simulink library "SpeedgoatModified"  (R2013a)
settings: Solver=ode45  StartTime=0.0  StopTime=60  RelTol=1e-3
undefined symbols (not defined in the file): standard
libraries: speedgoatlib x25, xpcseriallib x6, simulink x4, xpclib x2
settings Model: Creator=bgbuss  LastModifiedBy=bgbuss

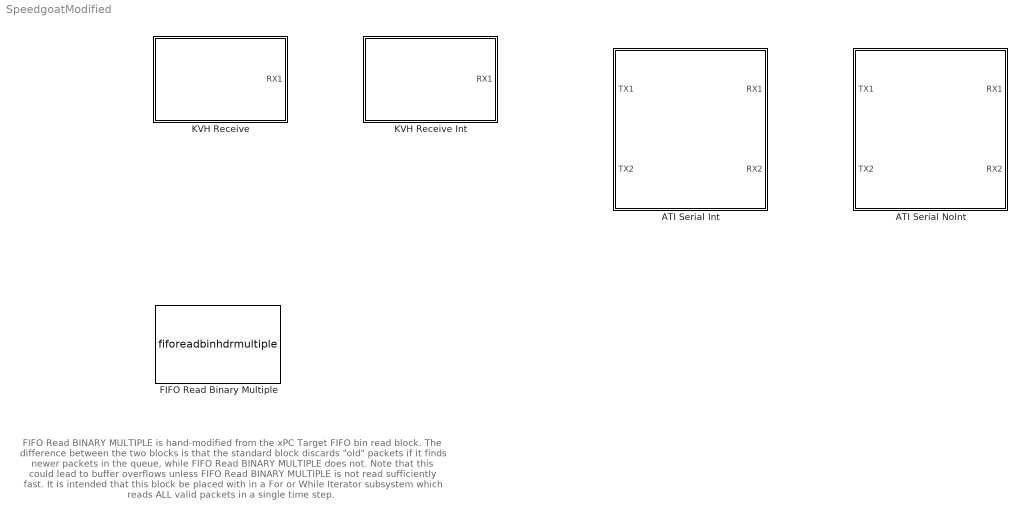
== system SpeedgoatModified ==
  note: FIFO Read BINARY MULTIPLE is hand-modified from the
      | xPC Target FIFO bin read block. The difference between the
      | two blocks is that the standard block discards "old" packets if it
      | finds newer packets in the queue, while FIFO Read BINARY MULTIPLE
      | does not. Note that this could lead to buffer overflows unless FIFO Read
      | BINARY MULTIPLE is not read sufficiently fast. It is intended that this block
      | be placed with in a For or While Iterator subsystem which reads ALL valid
      | packets in a single time step.
  ATI Serial Int : Subsystem
      mask Display:
      | disp('IO503\nTPMC466\nSend Interrupt-Free\nReceive Interrup-Driven')
      | 
      | port_label('input', 1, 'TX1')
      | port_label('input', 2, 'TX2')
      | 
      | port_label('output', 1, 'RX1')
      | port_label('output', 2, 'RX2')
  ATI Serial NoInt : Subsystem
      mask Display:
      | disp('IO503\nTPMC466\nSend Interrupt-Free\nReceive Interrup-Free')
      | 
      | port_label('input', 1, 'TX1')
      | port_label('input', 2, 'TX2')
      | 
      | port_label('output', 1, 'RX1')
      | port_label('output', 2, 'RX2')
  FIFO Read Binary Multiple : S-Function  FunctionName=fiforeadbinhdrmultiple  Parameters=maxsize, outputtype, sampletime, hdr, hlengths, lengths, hold, enable  EnableBusSupport=off  mask(Asynchronous FIFO Block: reader){header={char([170, 1]), char([170,2])}, lengths=[3 4], hold=Zero output if no new data, enable=off, maxsize=1024, outputtype=8 bit uint null terminated, sampletime=0.01}
      mask prompts: lengths "Message Lengths:"; hold "Output behavior:"; enable "Enable input:"; maxsize "Maximum read size:"; outputtype "Output vector type:"
      mask help: FIFO read multiple binary headers
      mask init:
      | [maskdisplay, hdr, hlengths] = mfifobinhdrmultiple( header, lengths );
      | set_param( gcb, 'MaskDisplay', maskdisplay );
      mask Help: eval('xpcdoc(''FIFO_binread'')');
      mask TypeOptions hold: Hold last output if no new data | Zero output if no new data
      mask TypeOptions outputtype: count+32 bit int | count+32 bit uint | count+16 bit int | count+16 bit uint | 8 bit int null terminated | 8 bit uint null terminated
      mask Display: disp( 'FIFO Read\nBINARY MULTIPLE');port_label('input',1,'F');port_label('output',1,'1');port_label('output',2,'2');
  KVH Receive : Subsystem
      mask Display:
      | disp('IO503\nTPMC466\nReceive\nInterrup-Free')
      | port_label('output', 1, 'RX1')
  KVH Receive Int : Subsystem
      mask Display:
      | disp('IO503\nTPMC466\nReceive\nInterrup-Driven')
      | port_label('output', 1, 'RX1')

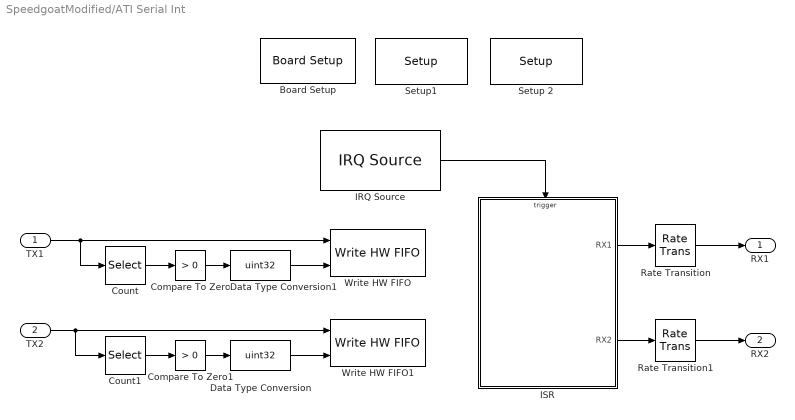
== system SpeedgoatModified/ATI Serial Int ==
  TX1 : Inport
  TX2 : Inport  Port=2
  Board Setup : speedgoatlib/IO503/TEWS TPMC466 Internal blocks/Board Setup  irqnum=5  slot=[4 4]
  Compare To Zero : simulink/Logic and Bit Operations/Compare To Zero  relop=>  OutDataTypeStr=uint8
  Compare To Zero1 : simulink/Logic and Bit Operations/Compare To Zero  relop=>  OutDataTypeStr=uint8
  Count : Selector  IndexMode=Zero-based  IndexOptions=Index vector (dialog)  Indices=0  OutputSizes=1
  Count1 : Selector  IndexMode=Zero-based  IndexOptions=Index vector (dialog)  Indices=0  OutputSizes=1
  Data Type Conversion : DataTypeConversion  OutDataTypeStr=uint32
  Data Type Conversion1 : DataTypeConversion  OutDataTypeStr=uint32
  IRQ Source : xpclib/Asynchronous Event/IRQ Source  irqNo=5  preempt=10  b_type=None/Other  slot=[4 4]
  ISR : Subsystem
  Rate Transition : RateTransition  Integrity=off  Deterministic=off
  Rate Transition1 : RateTransition  Integrity=off  Deterministic=off
  Setup 2 : speedgoatlib/IO503/TEWS TPMC466 Internal blocks/Setup   port=2  transceiver=RS485 half-duplex  standard=on  baudrate=1382400  bauddivisor=1  mode8x=16x (standard)  prescale=off  width=8  nstop=1  parity=Even  rlevel=half full (32)  ctsmode=none  xonoff=none  xon=17  xoff=19  rs485mode=on  rs485delay=0  slot=[4 4]
  "Setup1 " : speedgoatlib/IO503/TEWS TPMC466 Internal blocks/Setup   port=1  transceiver=RS485 half-duplex  standard=on  baudrate=1382400  bauddivisor=1  mode8x=16x (standard)  prescale=off  width=8  nstop=1  parity=Even  rlevel=half full (32)  ctsmode=none  xonoff=none  xon=17  xoff=19  rs485mode=on  rs485delay=0  slot=[4 4]
  Write HW FIFO : speedgoatlib/IO503/TEWS TPMC466 Internal blocks/Write HW FIFO  port=1  slot=[4 4]
  Write HW FIFO1 : speedgoatlib/IO503/TEWS TPMC466 Internal blocks/Write HW FIFO  port=2  slot=[4 4]
  RX1 : Outport
  RX2 : Outport  Port=2
  wires:
  Data Type Conversion1/1 -> Write HW FIFO/2
  Data Type Conversion/1 -> Write HW FIFO1/2
  Rate Transition/1 -> RX1/1
  IRQ Source/1 -> ISR/Trigger
  ISR/1(RX1) -> Rate Transition/1
  Rate Transition1/1 -> RX2/1
  ISR/2(RX2) -> Rate Transition1/1
  TX1/1 -> Count/1, Write HW FIFO/1
  TX2/1 -> Count1/1, Write HW FIFO1/1
  Count/1 -> Compare To Zero/1
  Count1/1 -> Compare To Zero1/1
  Compare To Zero1/1 -> Data Type Conversion/1
  Compare To Zero/1 -> Data Type Conversion1/1

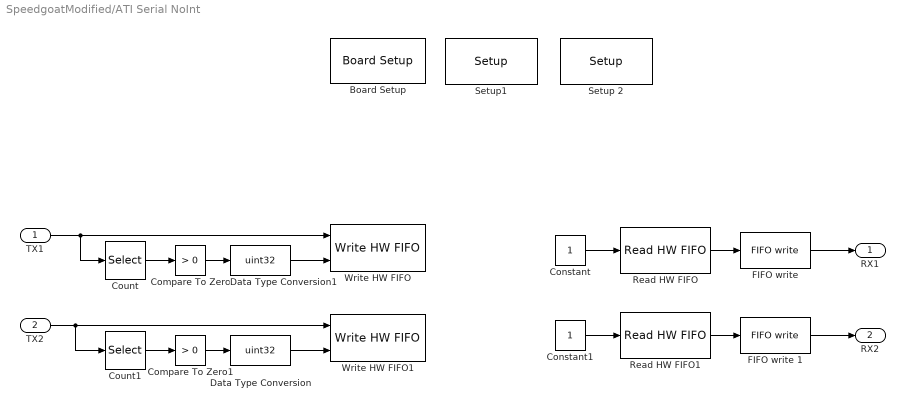
== system SpeedgoatModified/ATI Serial NoInt ==
  TX1 : Inport
  TX2 : Inport  Port=2
  Board Setup : speedgoatlib/IO503/TEWS TPMC466 Internal blocks/Board Setup  irqnum=5  slot=[4 4]
  Compare To Zero : simulink/Logic and Bit Operations/Compare To Zero  relop=>  OutDataTypeStr=uint8
  Compare To Zero1 : simulink/Logic and Bit Operations/Compare To Zero  relop=>  OutDataTypeStr=uint8
  Constant : Constant  OutDataTypeStr=Inherit: Inherit via back propagation
  Constant1 : Constant  OutDataTypeStr=Inherit: Inherit via back propagation
  Count : Selector  IndexMode=Zero-based  IndexOptions=Index vector (dialog)  Indices=0  OutputSizes=1
  Count1 : Selector  IndexMode=Zero-based  IndexOptions=Index vector (dialog)  Indices=0  OutputSizes=1
  Data Type Conversion : DataTypeConversion  OutDataTypeStr=uint32
  Data Type Conversion1 : DataTypeConversion  OutDataTypeStr=uint32
  "FIFO write " : xpcseriallib/FIFO write   size=256  inputtype=count+32 bit uint  present=off  sampletime=-1  id=IO503: IRQ 5 PCI Bus 4 Slot 4 (ATI F/T) 1
  FIFO write 1 : xpcseriallib/FIFO write   size=256  inputtype=count+32 bit uint  present=off  sampletime=-1  id=IO503: IRQ 5 PCI Bus 4 Slot 4 (ATI F/T) 2
  Read HW FIFO : speedgoatlib/IO503/TEWS TPMC466 Internal blocks/Read HW FIFO  port=1  flush=off  slot=[4 4]
  Read HW FIFO1 : speedgoatlib/IO503/TEWS TPMC466 Internal blocks/Read HW FIFO  port=2  flush=off  slot=[4 4]
  Setup 2 : speedgoatlib/IO503/TEWS TPMC466 Internal blocks/Setup   port=2  transceiver=RS485 half-duplex  standard=on  baudrate=1382400  bauddivisor=1  mode8x=16x (standard)  prescale=off  width=8  nstop=1  parity=Even  rlevel=almost full (56)  ctsmode=none  xonoff=none  xon=17  xoff=19  rs485mode=on  rs485delay=0  slot=[4 4]
  "Setup1 " : speedgoatlib/IO503/TEWS TPMC466 Internal blocks/Setup   port=1  transceiver=RS485 half-duplex  standard=on  baudrate=1382400  bauddivisor=1  mode8x=16x (standard)  prescale=off  width=8  nstop=1  parity=Even  rlevel=almost full (56)  ctsmode=none  xonoff=none  xon=17  xoff=19  rs485mode=on  rs485delay=0  slot=[4 4]
  Write HW FIFO : speedgoatlib/IO503/TEWS TPMC466 Internal blocks/Write HW FIFO  port=1  slot=[4 4]
  Write HW FIFO1 : speedgoatlib/IO503/TEWS TPMC466 Internal blocks/Write HW FIFO  port=2  slot=[4 4]
  RX1 : Outport  SourceOfInitialOutputValue=Input signal
  RX2 : Outport  Port=2  SourceOfInitialOutputValue=Input signal
  wires:
  Compare To Zero/1 -> Data Type Conversion1/1
  Compare To Zero1/1 -> Data Type Conversion/1
  Count1/1 -> Compare To Zero1/1
  Count/1 -> Compare To Zero/1
  TX2/1 -> Write HW FIFO1/1, Count1/1
  TX1/1 -> Write HW FIFO/1, Count/1
  Data Type Conversion/1 -> Write HW FIFO1/2
  Data Type Conversion1/1 -> Write HW FIFO/2
  Read HW FIFO1/1 -> FIFO write 1/1
  Constant1/1 -> Read HW FIFO1/1
  FIFO write 1/1 -> RX2/1
  Read HW FIFO/1 -> "FIFO write "/1
  Constant/1 -> Read HW FIFO/1
  "FIFO write "/1 -> RX1/1

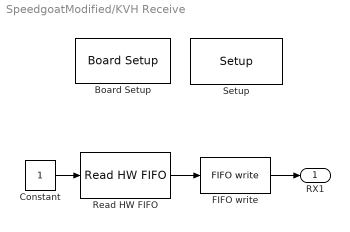
== system SpeedgoatModified/KVH Receive ==
  Board Setup : speedgoatlib/IO503/TEWS TPMC466 Internal blocks/Board Setup  irqnum=9  slot=[4 5]
  Constant : Constant  OutDataTypeStr=uint32
  "FIFO write " : xpcseriallib/FIFO write   size=256  inputtype=count+32 bit uint  present=off  sampletime=-1  id=IO503: IRQ 9 PCI Bus 4 Slot 5 (KVH IMU)
  Read HW FIFO : speedgoatlib/IO503/TEWS TPMC466 Internal blocks/Read HW FIFO  port=1  flush=off  slot=[4 5]
  "Setup " : speedgoatlib/IO503/TEWS TPMC466 Internal blocks/Setup   port=1  transceiver=RS422  standard=on  baudrate=921600  bauddivisor=1  mode8x=16x (standard)  prescale=off  width=8  nstop=1  parity=None  rlevel=almost full (56)  ctsmode=none  xonoff=none  xon=17  xoff=19  rs485mode=off  rs485delay=0  slot=[4 5]
  RX1 : Outport
  wires:
  Read HW FIFO/1 -> "FIFO write "/1
  "FIFO write "/1 -> RX1/1
  Constant/1 -> Read HW FIFO/1

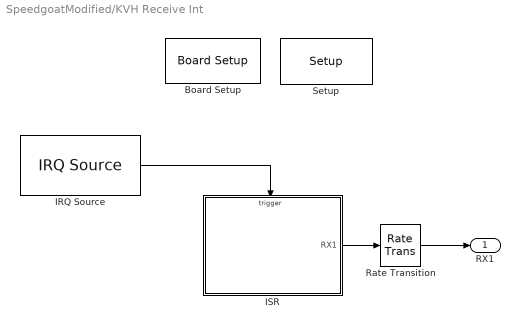
== system SpeedgoatModified/KVH Receive Int ==
  Board Setup : speedgoatlib/IO503/TEWS TPMC466 Internal blocks/Board Setup  irqnum=9  slot=[4 5]
  IRQ Source : xpclib/Asynchronous Event/IRQ Source  irqNo=9  preempt=10  b_type=None/Other  slot=[4 5]
  ISR : Subsystem
  Rate Transition : RateTransition  Integrity=off  Deterministic=off
  "Setup " : speedgoatlib/IO503/TEWS TPMC466 Internal blocks/Setup   port=1  transceiver=RS422  standard=on  baudrate=921600  bauddivisor=1  mode8x=16x (standard)  prescale=off  width=8  nstop=1  parity=None  rlevel=almost full (56)  ctsmode=none  xonoff=none  xon=17  xoff=19  rs485mode=off  rs485delay=0  slot=[4 5]
  RX1 : Outport
  wires:
  ISR/1(RX1) -> Rate Transition/1
  IRQ Source/1 -> ISR/Trigger
  Rate Transition/1 -> RX1/1

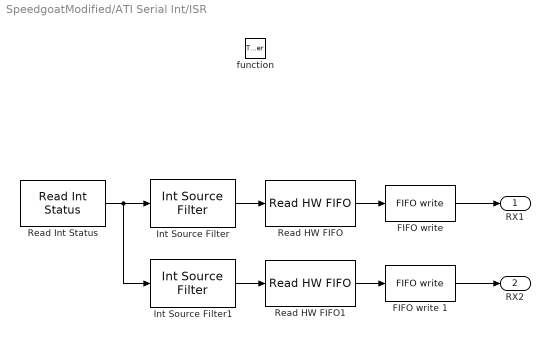
== system SpeedgoatModified/ATI Serial Int/ISR ==
  function : TriggerPort  TriggerType=function-call
  "FIFO write " : xpcseriallib/FIFO write   size=256  inputtype=count+32 bit uint  present=off  sampletime=-1  id=IO503: IRQ 5 PCI Bus 4 Slot 4 (ATI F/T) 1
  FIFO write 1 : xpcseriallib/FIFO write   size=256  inputtype=count+32 bit uint  present=off  sampletime=-1  id=IO503: IRQ 5 PCI Bus 4 Slot 4 (ATI F/T) 2
  Int Source Filter : speedgoatlib/IO503/TEWS TPMC466 Internal blocks/Int Source Filter  port=1  value=Receive data
  Int Source Filter1 : speedgoatlib/IO503/TEWS TPMC466 Internal blocks/Int Source Filter  port=2  value=Receive data
  Read HW FIFO : speedgoatlib/IO503/TEWS TPMC466 Internal blocks/Read HW FIFO  port=1  flush=off  slot=[4 4]
  Read HW FIFO1 : speedgoatlib/IO503/TEWS TPMC466 Internal blocks/Read HW FIFO  port=2  flush=off  slot=[4 4]
  Read Int Status : speedgoatlib/IO503/TEWS TPMC466 Internal blocks/Read Int Status  slot=[4 4]
  RX1 : Outport  SourceOfInitialOutputValue=Input signal
  RX2 : Outport  Port=2  SourceOfInitialOutputValue=Input signal
  wires:
  "FIFO write "/1 -> RX1/1
  Int Source Filter/1 -> Read HW FIFO/1
  Read Int Status/1 -> Int Source Filter1/1, Int Source Filter/1
  Read HW FIFO/1 -> "FIFO write "/1
  FIFO write 1/1 -> RX2/1
  Int Source Filter1/1 -> Read HW FIFO1/1
  Read HW FIFO1/1 -> FIFO write 1/1

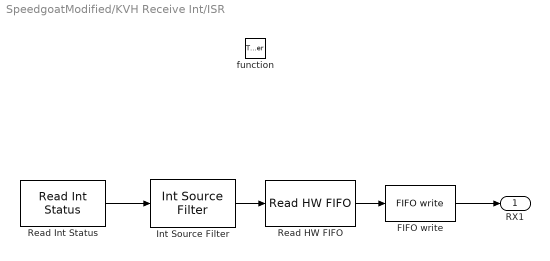
== system SpeedgoatModified/KVH Receive Int/ISR ==
  function : TriggerPort  TriggerType=function-call
  "FIFO write " : xpcseriallib/FIFO write   size=256  inputtype=count+32 bit uint  present=off  sampletime=-1  id=IO503: IRQ 9 PCI Bus 4 Slot 5 (KVH IMU)
  Int Source Filter : speedgoatlib/IO503/TEWS TPMC466 Internal blocks/Int Source Filter  port=1  value=Receive data
  Read HW FIFO : speedgoatlib/IO503/TEWS TPMC466 Internal blocks/Read HW FIFO  port=1  flush=off  slot=[4 5]
  Read Int Status : speedgoatlib/IO503/TEWS TPMC466 Internal blocks/Read Int Status  slot=[4 5]
  RX1 : Outport  SourceOfInitialOutputValue=Input signal
  wires:
  Read HW FIFO/1 -> "FIFO write "/1
  Read Int Status/1 -> Int Source Filter/1
  Int Source Filter/1 -> Read HW FIFO/1
  "FIFO write "/1 -> RX1/1
